simulink model "six_plus_six_AcmsteeringV09_main_1lf"  (R2014a)
settings: Solver=FixedStepDiscrete  StartTime=0.0  StopTime=10.0  FixedStep=0.0005  RelTol=1e-3
InitFcn:
  | Veh_Par_wxt
undefined symbols (not defined in the file or in its folder): acc_spdctl, ag_thr, B, bra_em, bra_pre_gz2, bra_pre_gz34, bra_pre_yd, brakepre_dem_data, brakeTrq_dem_data, bratrq_max, ecucoder_acal, eff_tran, ESP_switch, G, guzhang_lf, guzhang_lm, guzhang_lr, guzhang_rf, guzhang_rm, guzhang_rr, kd1, kd2, ki1, ki2, kp1, kp2, L, myFIS, premax, Radius, RC_switch, s_opt_yi, s_opt_zhuan, s_opt_zhuan_add, s_opt_zhuan_table, spd_map_mot, spd_spdctl, speed_thr_park, TCS_switch, tras_ratio, trq_map_mot, trqmax_yd, trqmax_zx, trqmaxneg, v_gain, v_table, v_thr_park, zhidong_bianmazhi, zhidong_down, zhidong_up, zhidong_youmen, zhuanxiang_bianmazhi, zhuanxiang_down, zhuanxiang_up, zhuanxiang_youmen
libraries: simulink x980, ec5744lib x59, fuzblock x2
(part 17 of 25)

== system six_plus_six_AcmsteeringV09_main_1lf/MainControl/mode_control/emergency_stop/emergency_stop ==
  Signals : Inport
  1-D Lookup Table : Lookup_n-D  NumberOfTableDimensions=1  BreakpointsForDimension1=zhuanxiang_youmen  Table=zhuanxiang_bianmazhi  InternalRulePriority=Speed  RndMeth=Simplest  InputSameDT=on
  1-D Lookup Table1 : Lookup_n-D  NumberOfTableDimensions=1  BreakpointsForDimension1=zhidong_youmen  Table=zhidong_bianmazhi  InternalRulePriority=Speed  RndMeth=Simplest  InputSameDT=on
  Bus Selector1 : BusSelector  OutputSignals=RemoteControl_dem.steer_dem
  Constant : Constant  Value=bra_em  OutDataTypeStr=single  SampleTime=-1
  Gain : Gain  Gain=0.5
  Gain1 : Gain  Gain=-1
  HeartBeat : MATLAB Function  TreatAsAtomicUnit=on
  HeartBeat1 : MATLAB Function  TreatAsAtomicUnit=on
  HeartBeat2 : MATLAB Function  TreatAsAtomicUnit=on
  HeartBeat3 : MATLAB Function  TreatAsAtomicUnit=on
  HeartBeat4 : MATLAB Function  TreatAsAtomicUnit=on
  HeartBeat5 : MATLAB Function  TreatAsAtomicUnit=on
  Memory{,1..4,6} (6 alike) : Memory  InheritSampleTime=on
  Mux{,1..5} (6 alike) : Mux  Inputs=6
  Saturation : Saturate  UpperLimit=zhuanxiang_up  LowerLimit=zhuanxiang_down
  Saturation2 : Saturate  UpperLimit=zhuanxiang_up  LowerLimit=zhuanxiang_down
  Saturation3 : Saturate  UpperLimit=zhuanxiang_up  LowerLimit=zhuanxiang_down
  Saturation5 : Saturate  UpperLimit=zhidong_up  LowerLimit=zhidong_down
  SpdSet_dem{,1..5} (6 alike) : Constant  Value=0  OutDataTypeStr=single  SampleTime=-1
  TrqSet_dem{,1..5} (6 alike) : Constant  Value=0  OutDataTypeStr=single  SampleTime=-1
  mot_enable{,1..5} (6 alike) : Constant  Value=0  OutDataTypeStr=single  SampleTime=-1
  mot_gear{,1..5} (6 alike) : Constant  Value=0  OutDataTypeStr=single  SampleTime=-1
  mot_mode{,1..5} (6 alike) : Constant  Value=0  OutDataTypeStr=single  SampleTime=-1
  mot_lf : Outport
  mot_lm : Outport  Port=2
  mot_lr : Outport  Port=3
  mot_rf : Outport  Port=4
  mot_rm : Outport  Port=5
  mot_rr : Outport  Port=6
  motec_position_1 : Outport  Port=7
  motec_position_2 : Outport  Port=8
  motec_position_3 : Outport  Port=9
  motec_position_4 : Outport  Port=10
  wires:
  mot_gear/1 -> Mux/3
  mot_mode/1 -> Mux/2
  SpdSet_dem/1 -> Mux/4
  TrqSet_dem/1 -> Mux/5
  Mux/1 -> mot_lf/1
  HeartBeat/1(life) -> Mux/6, Memory/1
  Memory/1 -> HeartBeat/1(life_pre)
  mot_enable/1 -> Mux/1
  mot_gear1/1 -> Mux2/3
  mot_mode2/1 -> Mux2/2
  SpdSet_dem1/1 -> Mux2/4
  TrqSet_dem1/1 -> Mux2/5
  Mux2/1 -> mot_rf/1
  HeartBeat2/1(life) -> Memory2/1, Mux2/6
  Memory2/1 -> HeartBeat2/1(life_pre)
  mot_enable1/1 -> Mux2/1
  mot_gear2/1 -> Mux4/3
  mot_mode4/1 -> Mux4/2
  SpdSet_dem4/1 -> Mux4/4
  TrqSet_dem4/1 -> Mux4/5
  Mux4/1 -> mot_lm/1
  HeartBeat3/1(life) -> Memory4/1, Mux4/6
  Memory4/1 -> HeartBeat3/1(life_pre)
  mot_enable3/1 -> Mux4/1
  mot_gear3/1 -> Mux5/3
  mot_mode5/1 -> Mux5/2
  SpdSet_dem5/1 -> Mux5/4
  TrqSet_dem5/1 -> Mux5/5
  Mux5/1 -> mot_rm/1
  HeartBeat4/1(life) -> Mux5/6, Memory6/1
  Memory6/1 -> HeartBeat4/1(life_pre)
  mot_enable5/1 -> Mux5/1
  mot_gear4/1 -> Mux1/3
  mot_mode1/1 -> Mux1/2
  SpdSet_dem2/1 -> Mux1/4
  TrqSet_dem2/1 -> Mux1/5
  Mux1/1 -> mot_lr/1
  HeartBeat1/1(life) -> Memory1/1, Mux1/6
  Memory1/1 -> HeartBeat1/1(life_pre)
  mot_enable4/1 -> Mux1/1
  mot_gear5/1 -> Mux3/3
  mot_mode3/1 -> Mux3/2
  SpdSet_dem3/1 -> Mux3/4
  TrqSet_dem3/1 -> Mux3/5
  Mux3/1 -> mot_rr/1
  HeartBeat5/1(life) -> Memory3/1, Mux3/6
  Memory3/1 -> HeartBeat5/1(life_pre)
  mot_enable2/1 -> Mux3/1
  1-D Lookup Table1/1 -> Saturation5/1
  1-D Lookup Table/1 -> Gain1/1, Gain/1, Saturation/1
  Signals/1 -> Bus Selector1/1
  Gain1/1 -> Saturation3/1
  Bus Selector1/1 -> 1-D Lookup Table/1  "<steer_dem>"
  Gain/1 -> Saturation2/1
  Saturation/1 -> motec_position_1/1
  Saturation2/1 -> motec_position_2/1
  Saturation3/1 -> motec_position_3/1
  Saturation5/1 -> motec_position_4/1
  Constant/1 -> 1-D Lookup Table1/1

== system six_plus_six_AcmsteeringV09_main_1lf/MainControl/mode_control/forward/forward ==
  Signals : Inport
  Brake : Subsystem  TreatAsAtomicUnit=on
  Bus Selector : BusSelector  OutputSignals=RemoteControl_dem.acc_dem,RemoteControl_dem.brake_dem,RemoteControl_dem.HAC
  Drive : Subsystem  TreatAsAtomicUnit=on
  MATLAB Function : MATLAB Function  TreatAsAtomicUnit=on
  Multiport Switch : MultiPortSwitch  DataPortOrder=Zero-based contiguous  Inputs=2
  Switch Case1 : SwitchCase  CaseConditions={0,1}  ShowDefaultCase=off
  forward_dem : Outport
  wires:
  Signals/1 -> Brake/1(Signals), Drive/1(Signals), Bus Selector/1
  Multiport Switch/1 -> forward_dem/1
  Switch Case1/1 -> Drive/Action
  Switch Case1/2 -> Brake/Action
  Bus Selector/1 -> MATLAB Function/1(acc_dem)  "<acc_dem>"
  MATLAB Function/1(y) -> Multiport Switch/1, Switch Case1/1
  Drive/1(forward_dem) -> Multiport Switch/2
  Brake/1(forward_dem) -> Multiport Switch/3
  Bus Selector/2 -> MATLAB Function/2(brake_dem)  "<brake_dem>"
  Bus Selector/3 -> MATLAB Function/3(HAC)  "<HAC>"

== matlab function six_plus_six_AcmsteeringV09_main_1lf/MainControl/mode_control/Park/park/HeartBeat3 ==
  data: life_pre input; life output
function life = fcn(life_pre)
%#codegen
life=single(life_pre+1);
if life>255
    life=single(0);
end
end

== system six_plus_six_AcmsteeringV09_main_1lf/MainControl/mode_control/neutral/neutral ==
  Signals : Inport
  1-D Lookup Table1 : Lookup_n-D  NumberOfTableDimensions=1  BreakpointsForDimension1=zhuanxiang_youmen  Table=zhuanxiang_bianmazhi  InternalRulePriority=Speed  RndMeth=Simplest  InputSameDT=on
  1-D Lookup Table2 : Lookup_n-D  NumberOfTableDimensions=1  BreakpointsForDimension1=zhidong_youmen  Table=zhidong_bianmazhi  InternalRulePriority=Speed  RndMeth=Simplest  InputSameDT=on
  Bus Selector : BusSelector  OutputSignals=RemoteControl_dem.steer_dem,RemoteControl_dem.brake_dem
  Gain : Gain  Gain=0.5
  Gain1 : Gain  Gain=-1
  HeartBeat : MATLAB Function  TreatAsAtomicUnit=on
  HeartBeat1 : MATLAB Function  TreatAsAtomicUnit=on
  HeartBeat2 : MATLAB Function  TreatAsAtomicUnit=on
  HeartBeat3 : MATLAB Function  TreatAsAtomicUnit=on
  HeartBeat4 : MATLAB Function  TreatAsAtomicUnit=on
  HeartBeat5 : MATLAB Function  TreatAsAtomicUnit=on
  Memory{,1..4,6} (6 alike) : Memory  InheritSampleTime=on
  Mux{,1..5} (6 alike) : Mux  Inputs=6
  Saturation : Saturate  UpperLimit=zhuanxiang_up  LowerLimit=zhuanxiang_down
  Saturation1 : Saturate  UpperLimit=zhuanxiang_up  LowerLimit=zhuanxiang_down
  Saturation2 : Saturate  UpperLimit=zhuanxiang_up  LowerLimit=zhuanxiang_down
  Saturation3 : Saturate  UpperLimit=zhidong_up  LowerLimit=zhidong_down
  SpdSet_dem{,1..5} (6 alike) : Constant  Value=0  OutDataTypeStr=single  SampleTime=-1
  TrqSet_dem{,1..5} (6 alike) : Constant  Value=0  OutDataTypeStr=single  SampleTime=-1
  mot_enable{,1..5} (6 alike) : Constant  Value=0  OutDataTypeStr=single  SampleTime=-1
  mot_gear{,1..5} (6 alike) : Constant  Value=0  OutDataTypeStr=single  SampleTime=-1
  mot_mode{,1..5} (6 alike) : Constant  Value=0  OutDataTypeStr=single  SampleTime=-1
  mot_lf : Outport
  mot_lm : Outport  Port=2
  mot_lr : Outport  Port=3
  mot_rf : Outport  Port=4
  mot_rm : Outport  Port=5
  mot_rr : Outport  Port=6
  motec_position_1 : Outport  Port=7
  motec_position_2 : Outport  Port=8
  motec_position_3 : Outport  Port=9
  motec_position_4 : Outport  Port=10
  wires:
  mot_gear/1 -> Mux/3
  mot_mode/1 -> Mux/2
  SpdSet_dem/1 -> Mux/4
  TrqSet_dem/1 -> Mux/5
  Mux/1 -> mot_lf/1
  HeartBeat/1(life) -> Mux/6, Memory/1
  Memory/1 -> HeartBeat/1(life_pre)
  mot_enable/1 -> Mux/1
  mot_gear1/1 -> Mux2/3
  mot_mode2/1 -> Mux2/2
  SpdSet_dem1/1 -> Mux2/4
  TrqSet_dem1/1 -> Mux2/5
  Mux2/1 -> mot_rf/1
  HeartBeat2/1(life) -> Memory2/1, Mux2/6
  Memory2/1 -> HeartBeat2/1(life_pre)
  mot_enable1/1 -> Mux2/1
  mot_gear2/1 -> Mux4/3
  mot_mode4/1 -> Mux4/2
  SpdSet_dem4/1 -> Mux4/4
  TrqSet_dem4/1 -> Mux4/5
  Mux4/1 -> mot_lm/1
  HeartBeat3/1(life) -> Memory4/1, Mux4/6
  Memory4/1 -> HeartBeat3/1(life_pre)
  mot_enable3/1 -> Mux4/1
  mot_gear3/1 -> Mux5/3
  mot_mode5/1 -> Mux5/2
  SpdSet_dem5/1 -> Mux5/4
  TrqSet_dem5/1 -> Mux5/5
  Mux5/1 -> mot_rm/1
  HeartBeat4/1(life) -> Mux5/6, Memory6/1
  Memory6/1 -> HeartBeat4/1(life_pre)
  mot_enable5/1 -> Mux5/1
  mot_gear4/1 -> Mux1/3
  mot_mode1/1 -> Mux1/2
  SpdSet_dem2/1 -> Mux1/4
  TrqSet_dem2/1 -> Mux1/5
  Mux1/1 -> mot_lr/1
  HeartBeat1/1(life) -> Memory1/1, Mux1/6
  Memory1/1 -> HeartBeat1/1(life_pre)
  mot_enable4/1 -> Mux1/1
  mot_gear5/1 -> Mux3/3
  mot_mode3/1 -> Mux3/2
  SpdSet_dem3/1 -> Mux3/4
  TrqSet_dem3/1 -> Mux3/5
  Mux3/1 -> mot_rr/1
  HeartBeat5/1(life) -> Memory3/1, Mux3/6
  Memory3/1 -> HeartBeat5/1(life_pre)
  mot_enable2/1 -> Mux3/1
  1-D Lookup Table1/1 -> Gain1/1, Gain/1, Saturation/1
  Signals/1 -> Bus Selector/1
  Gain1/1 -> Saturation2/1
  Bus Selector/1 -> 1-D Lookup Table1/1  "<steer_dem>"
  Gain/1 -> Saturation1/1
  Saturation/1 -> motec_position_1/1
  Saturation1/1 -> motec_position_2/1
  Saturation2/1 -> motec_position_3/1
  Saturation3/1 -> motec_position_4/1
  Bus Selector/2 -> 1-D Lookup Table2/1  "<brake_dem>"
  1-D Lookup Table2/1 -> Saturation3/1

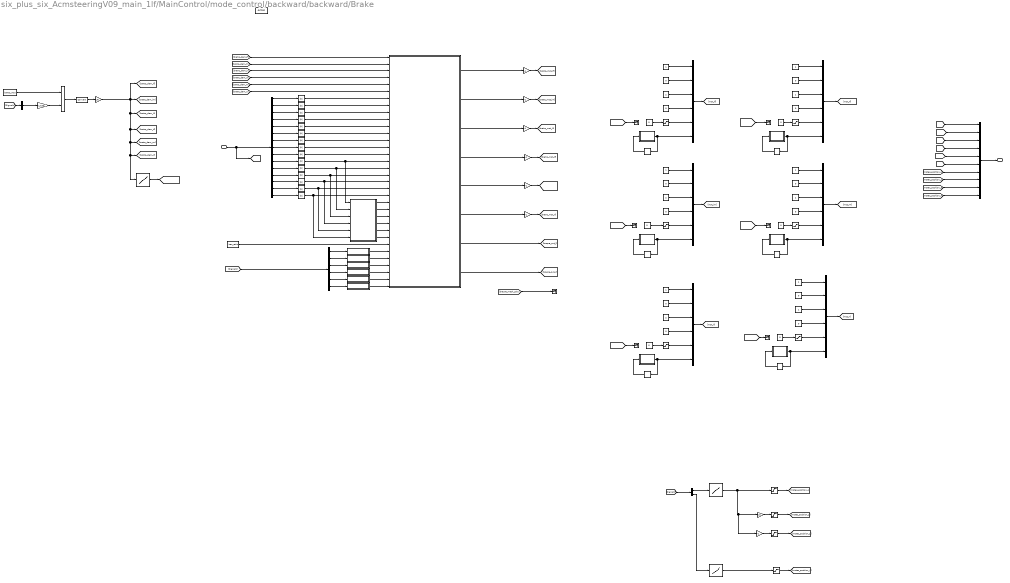
== system six_plus_six_AcmsteeringV09_main_1lf/MainControl/mode_control/backward/backward/Brake ==
  note: 当时编程序时候，fcn里面正负号搞错了，不得已在外面乘以-1，
      | 当制动时，电池功率限制，电机扭矩限制当做正值处理，电机
      | 输出力矩也是正值
  note: 制动力矩四个车轮平均分配
  Signals : Inport
  Action Port : ActionPort  ActionType=case
  1-D Lookup Table : Lookup_n-D  NumberOfTableDimensions=1  BreakpointsForDimension1=brakeTrq_dem_data  Table=brakepre_dem_data  InternalRulePriority=Speed  RndMeth=Simplest  InputSameDT=on
  1-D Lookup Table1 : Lookup_n-D  NumberOfTableDimensions=1  BreakpointsForDimension1=zhuanxiang_youmen  Table=zhuanxiang_bianmazhi  InternalRulePriority=Speed  RndMeth=Simplest  InputSameDT=on
  1-D Lookup Table2 : Lookup_n-D  NumberOfTableDimensions=1  BreakpointsForDimension1=zhidong_youmen  Table=zhidong_bianmazhi  InternalRulePriority=Speed  RndMeth=Simplest  InputSameDT=on
  Abs{1..5,10..19} (15 alike) : Abs  OutDataTypeStr=single
  Bus Selector : BusSelector  OutputSignals=RemoteControl_dem.steer_dem,RemoteControl_dem.brake_dem
  Bus Selector1 : BusSelector  OutputSignals=MOTOR.MOTOR1.MCU2,MOTOR.MOTOR3.MCU2-2,MOTOR.MOTOR5.MCU2_4,MOTOR.MOTOR2.MCU2_1,MOTOR.MOTOR4.MCU2_3,MOTOR.MOTOR6.MCU2_5
  Bus Selector2 : BusSelector  OutputSignals=RemoteControl_dem.brake_dem
  Bus Selector3 : BusSelector  OutputSignals=CCM.CCM1.BMS5.BMS5_FeedbackPower,CCM.CCM2.BMS5_1.BMS5_1FeedbackPower,CCM.CCM3.BMS5_2.BMS5_2FeedbackPower,MOTOR.MOTOR1.MCU0.MCU0_TorqueMax,MOTOR.MOTOR3.MCU0_2.MCU0_2TorqueMax,MOTOR.MOTOR5.MCU0_4.MCU0_4TorqueMax,MOTOR.MOTOR2.MCU0_1.MCU0_1TorqueMax,MOTOR.MOTOR4.MCU0_3.MCU0_3TorqueMax,MOTOR.MOTOR6.MCU0_5.MCU0_5TorqueMax,MOTOR.MOTOR1.MCU0.MCU0_SpeedFdk,MOTOR.MOTOR3.MCU0_2.MCU0_2SpeedFdk,MOTOR.MOTOR5.MCU0_4.MCU0_4SpeedFdk,MOTOR.MOTOR2.MCU0_1.MCU0_1SpeedFdk,MOTOR.MOTOR4.MCU0_3.MCU0_3SpeedFdk,MOTOR.MOTOR6.MCU0_5.MCU0_5SpeedFdk
  Constant{,1..3,5..6} (6 alike) : Constant  Value=0  SampleTime=-1
  Constant4 : Constant  Value=bratrq_max  OutDataTypeStr=single  SampleTime=-1
  Constant7 : Constant  Value=tras_ratio  OutDataTypeStr=single  SampleTime=-1
  Data Type Conversion1 : DataTypeConversion
  Gain : Gain  Gain=1/6
  Gain1 : Gain  Gain=0.5
  Gain{3,7..10,15..16} (7 alike) : Gain  Gain=-1
  Gain2 : Gain  Gain=1/100
  HeartBeat : MATLAB Function  TreatAsAtomicUnit=on
  HeartBeat1 : MATLAB Function  TreatAsAtomicUnit=on
  HeartBeat2 : MATLAB Function  TreatAsAtomicUnit=on
  HeartBeat3 : MATLAB Function  TreatAsAtomicUnit=on
  HeartBeat4 : MATLAB Function  TreatAsAtomicUnit=on
  HeartBeat5 : MATLAB Function  TreatAsAtomicUnit=on
  Memory{1..6} (6 alike) : Memory  InheritSampleTime=on
  Mux : Mux  Inputs=10
  Mux{1..6} (6 alike) : Mux  Inputs=6
  Product : Product
  Saturation{,1..5} (6 alike) : Saturate  UpperLimit=0  LowerLimit=trqmaxneg  OutDataTypeStr=single
  Saturation10 : Saturate  UpperLimit=zhuanxiang_up  LowerLimit=zhuanxiang_down
  Saturation11 : Saturate  UpperLimit=zhidong_up  LowerLimit=zhidong_down
  Saturation8 : Saturate  UpperLimit=zhuanxiang_up  LowerLimit=zhuanxiang_down
  Saturation9 : Saturate  UpperLimit=zhuanxiang_up  LowerLimit=zhuanxiang_down
  SpdSet_dem{,1..5} (6 alike) : Constant  Value=0  OutDataTypeStr=single  SampleTime=-1
  Subsystem : Subsystem
  Subsystem1 : Subsystem
  Subsystem2 : Subsystem
  Subsystem3 : Subsystem
  Subsystem4 : Subsystem
  Subsystem5 : Subsystem
  Subsystem6 : Subsystem
  Switch Case Action Subsystem : Subsystem  TreatAsAtomicUnit=on
  Terminator{,1..6} (7 alike) : Terminator
  mot_enable{1..6} (6 alike) : Constant  OutDataTypeStr=single  SampleTime=-1
  mot_gear : Constant  Value=2  OutDataTypeStr=single  SampleTime=-1
  mot_gear1 : Constant  OutDataTypeStr=single  SampleTime=-1
  mot_gear2 : Constant  Value=2  OutDataTypeStr=single  SampleTime=-1
  mot_gear3 : Constant  OutDataTypeStr=single  SampleTime=-1
  mot_gear4 : Constant  Value=2  OutDataTypeStr=single  SampleTime=-1
  mot_gear5 : Constant  OutDataTypeStr=single  SampleTime=-1
  mot_mode{,1..5} (6 alike) : Constant  Value=0  OutDataTypeStr=single  SampleTime=-1
  backward_dem : Outport
  wires:
  [Signals] -> Bus Selector2/1
  Gain/1 -> [bratrq_dem_lm], [bratrq_dem_rm], 1-D Lookup Table/1, [bratrq_dem_rr], [bratrq_dem_rf], [bratrq_dem_lr], [bratrq_dem_lf]
  Memory4/1 -> HeartBeat/1(life_pre)
  HeartBeat/1(life) -> Mux1/6, Memory4/1
  Mux1/1 -> [mot_lf]
  mot_mode/1 -> Mux1/2
  mot_gear/1 -> Mux1/3
  [mot_lf] -> Mux/1
  Signals/1 -> [Signals], Bus Selector3/1
  Constant4/1 -> Product/1
  Gain2/1 -> Product/2
  Bus Selector2/1 -> Gain2/1  "<brake_dem>"
  Product/1 -> Data Type Conversion1/1
  Gain8/1 -> [bratrq_mot_lf]
  Gain7/1 -> [bratrq_mot_lr]
  Gain9/1 -> [bratrq_mot_rf]
  Gain10/1 -> [bratrq_mot_rr]
  Constant7/1 -> Switch Case Action Subsystem/28(tras_ratio)
  1-D Lookup Table/1 -> [brapre_mech_solo]
  Data Type Conversion1/1 -> Gain/1
  Mux/1 -> backward_dem/1
  [brapre_mech_solo] -> Terminator1/1
  Switch Case Action Subsystem/1(bratrq_mot_lf) -> Gain8/1
  Gain15/1 -> [bratrq_mot_lm]
  Switch Case Action Subsystem/2(bratrq_mot_lm) -> Gain15/1
  Switch Case Action Subsystem/3(bratrq_mot_lr) -> Gain7/1
  Switch Case Action Subsystem/4(bratrq_mot_rf) -> Gain9/1
  Gain16/1 -> [bratrq_mot_rm]
  Switch Case Action Subsystem/5(bratrq_mot_rm) -> Gain16/1
  Switch Case Action Subsystem/6(bratrq_mot_rr) -> Gain10/1
  Switch Case Action Subsystem/7(brapre_out_l) -> [brapre_out_l]
  Switch Case Action Subsystem/8(brapre_out_r) -> [brapre_out_r]
  [bratrq_dem_lf] -> Switch Case Action Subsystem/1(bratrq_dem_lf)
  [bratrq_dem_rf] -> Switch Case Action Subsystem/4(bratrq_dem_rf)
  [bratrq_dem_rr] -> Switch Case Action Subsystem/6(bratrq_dem_rr)
  [bratrq_dem_lr] -> Switch Case Action Subsystem/3(bratrq_dem_lr)
  [bratrq_dem_rm] -> Switch Case Action Subsystem/5(bratrq_dem_rm)
  [bratrq_dem_lm] -> Switch Case Action Subsystem/2(bratrq_dem_lm)
  Bus Selector3/1 -> Abs5/1  "<BMS5_FeedbackPower>"
  Bus Selector3/2 -> Abs1/1  "<BMS5_1FeedbackPower>"
  Bus Selector3/3 -> Abs2/1  "<BMS5_2FeedbackPower>"
  Bus Selector3/10 -> Abs14/1  "<MCU0_SpeedFdk>"
  Bus Selector3/5 -> Abs4/1  "<MCU0_2TorqueMax>"
  Bus Selector3/7 -> Abs11/1  "<MCU0_1TorqueMax>"
  Bus Selector3/6 -> Abs10/1  "<MCU0_4TorqueMax>"
  Bus Selector3/8 -> Abs12/1  "<MCU0_3TorqueMax>"
  Bus Selector3/9 -> Abs13/1  "<MCU0_5TorqueMax>"
  Bus Selector3/4 -> Abs3/1  "<MCU0_TorqueMax>"
  Bus Selector3/11 -> Abs15/1  "<MCU0_2SpeedFdk>"
  Bus Selector3/14 -> Abs18/1  "<MCU0_3SpeedFdk>"
  Bus Selector3/12 -> Abs16/1  "<MCU0_4SpeedFdk>"
  Bus Selector3/15 -> Abs19/1  "<MCU0_5SpeedFdk>"
  Bus Selector3/13 -> Abs17/1  "<MCU0_1SpeedFdk>"
  Abs5/1 -> Switch Case Action Subsystem/7(pwr_chg_bat)
  Abs1/1 -> Switch Case Action Subsystem/8(pwr_chg_bat1)
  Abs2/1 -> Switch Case Action Subsystem/9(pwr_chg_bat2)
  Abs3/1 -> Switch Case Action Subsystem/10(trqlimL_dig_lf)
  Abs4/1 -> Switch Case Action Subsystem/11(trqlimL_dig_lm)
  Abs10/1 -> Switch Case Action Subsystem/12(trqlimL_dig_lr)
  Abs11/1 -> Switch Case Action Subsystem/13(trqlimL_dig_rf)
  Abs12/1 -> Switch Case Action Subsystem/14(trqlimL_dig_rm)
  Abs13/1 -> Switch Case Action Subsystem/15(trqlimL_dig_rr)
  Abs14/1 -> Subsystem1/1(speed_act_lf), Switch Case Action Subsystem/16(speed_act_lf)
  Abs15/1 -> Subsystem1/2(speed_act_lm), Switch Case Action Subsystem/17(speed_act_lm)
  Abs16/1 -> Subsystem1/3(speed_act_lr), Switch Case Action Subsystem/18(speed_act_lr)
  Abs17/1 -> Subsystem1/4(speed_act_rf), Switch Case Action Subsystem/19(speed_act_rf)
  Abs18/1 -> Subsystem1/5(speed_act_rm), Switch Case Action Subsystem/20(speed_act_rm)
  Abs19/1 -> Subsystem1/6(speed_act_rr), Switch Case Action Subsystem/21(speed_act_rr)
  Subsystem1/1(trqlim_map_lf) -> Switch Case Action Subsystem/22(trqlim_map_lf)
  Subsystem1/2(trqlim_map_lm) -> Switch Case Action Subsystem/23(trqlim_map_lm)
  Subsystem1/3(trqlim_map_lr) -> Switch Case Action Subsystem/24(trqlim_map_lr)
  Subsystem1/4(trqlim_map_rf) -> Switch Case Action Subsystem/25(trqlim_map_rf)
  Subsystem1/5(trqlim_map_rm) -> Switch Case Action Subsystem/26(trqlim_map_rm)
  Subsystem1/6(trqlim_map_rr) -> Switch Case Action Subsystem/27(trqlim_map_rr)
  [Signals] -> Bus Selector1/1
  Bus Selector1/1 -> Subsystem/1(MCU2)  "<MCU2>"
  Subsystem/1(guzhang_lf) -> Switch Case Action Subsystem/29(guzhang_lf)
  Bus Selector1/2 -> Subsystem2/1(MCU2_2)  "<MCU2-2>"
  Subsystem2/1(guzhang_lm) -> Switch Case Action Subsystem/30(guzhang_lm)
  Bus Selector1/3 -> Subsystem3/1(MCU2_4)  "<MCU2_4>"
  Subsystem3/1(guzhang_lr) -> Switch Case Action Subsystem/31(guzhang_lr)
  Bus Selector1/4 -> Subsystem4/1(MCU2_1)  "<MCU2_1>"
  Subsystem4/1(guzhang_rf) -> Switch Case Action Subsystem/32(guzhang_rf)
  Bus Selector1/5 -> Subsystem5/1(MCU2_3)  "<MCU2_3>"
  Subsystem5/1(guzhang_rm) -> Switch Case Action Subsystem/33(guzhang_rm)
  Bus Selector1/6 -> Subsystem6/1(MCU2_5)  "<MCU2_5>"
  Subsystem6/1(guzhang_rr) -> Switch Case Action Subsystem/34(guzhang_rr)
  mot_enable4/1 -> Mux1/1
  [bratrq_mot_lf] -> Terminator/1
  SpdSet_dem/1 -> Mux1/4
  Saturation/1 -> Mux1/5
  Memory1/1 -> HeartBeat2/1(life_pre)
  HeartBeat2/1(life) -> Memory1/1, Mux3/6
  Mux3/1 -> [mot_rf]
  mot_mode2/1 -> Mux3/2
  mot_gear1/1 -> Mux3/3
  mot_enable2/1 -> Mux3/1
  SpdSet_dem1/1 -> Mux3/4
  Saturation2/1 -> Mux3/5
  Memory3/1 -> HeartBeat3/1(life_pre)
  HeartBeat3/1(life) -> Memory3/1, Mux5/6
  Mux5/1 -> [mot_lm]
  mot_mode4/1 -> Mux5/2
  mot_gear2/1 -> Mux5/3
  mot_enable6/1 -> Mux5/1
  SpdSet_dem4/1 -> Mux5/4
  Saturation4/1 -> Mux5/5
  Memory2/1 -> HeartBeat4/1(life_pre)
  HeartBeat4/1(life) -> Mux6/6, Memory2/1
  Mux6/1 -> [mot_rm]
  mot_mode5/1 -> Mux6/2
  mot_gear3/1 -> Mux6/3
  mot_enable5/1 -> Mux6/1
  SpdSet_dem5/1 -> Mux6/4
  Saturation5/1 -> Mux6/5
  Memory5/1 -> HeartBeat1/1(life_pre)
  HeartBeat1/1(life) -> Memory5/1, Mux2/6
  Mux2/1 -> [mot_lr]
  mot_mode1/1 -> Mux2/2
  mot_gear4/1 -> Mux2/3
  mot_enable1/1 -> Mux2/1
  SpdSet_dem2/1 -> Mux2/4
  Saturation1/1 -> Mux2/5
  Memory6/1 -> HeartBeat5/1(life_pre)
  HeartBeat5/1(life) -> Mux4/6, Memory6/1
  Mux4/1 -> [mot_rr]
  mot_mode3/1 -> Mux4/2
  mot_gear5/1 -> Mux4/3
  mot_enable3/1 -> Mux4/1
  SpdSet_dem3/1 -> Mux4/4
  Saturation3/1 -> Mux4/5
  [mot_lm] -> Mux/2
  [mot_lr] -> Mux/3
  [mot_rf] -> Mux/4
  [mot_rm] -> Mux/5
  [mot_rr] -> Mux/6
  [motec_position_1] -> Mux/7
  [motec_position_2] -> Mux/8
  [motec_position_3] -> Mux/9
  Constant/1 -> Saturation/1
  [bratrq_mot_lm] -> Terminator2/1
  Constant1/1 -> Saturation4/1
  [bratrq_mot_lr] -> Terminator3/1
  Constant2/1 -> Saturation1/1
  [bratrq_mot_rf] -> Terminator4/1
  Constant3/1 -> Saturation2/1
  [bratrq_mot_rm] -> Terminator5/1
  Constant5/1 -> Saturation5/1
  [bratrq_mot_rr] -> Terminator6/1
  Constant6/1 -> Saturation3/1
  1-D Lookup Table2/1 -> Saturation11/1
  1-D Lookup Table1/1 -> Gain3/1, Gain1/1, Saturation8/1
  [Signals] -> Bus Selector/1
  Gain3/1 -> Saturation10/1
  Bus Selector/1 -> 1-D Lookup Table1/1  "<steer_dem>"
  Gain1/1 -> Saturation9/1
  Saturation8/1 -> [motec_position_1]
  Saturation9/1 -> [motec_position_2]
  Saturation10/1 -> [motec_position_3]
  Saturation11/1 -> [motec_position_4]
  Bus Selector/2 -> 1-D Lookup Table2/1  "<brake_dem>"
  [motec_position_4] -> Mux/10

== system six_plus_six_AcmsteeringV09_main_1lf/MainControl/mode_control/backward/backward/Drive ==
  Signals : Inport
  Action Port : ActionPort  ActionType=case
  Abs{,1..24} (25 alike) : Abs  OutDataTypeStr=single
  Abs25 : Abs
  Bus Selector : BusSelector  OutputSignals=RemoteControl_dem.acc_dem,MOTOR.MOTOR1.MCU0.MCU0_TorqueMax,MOTOR.MOTOR3.MCU0_2.MCU0_2TorqueMax,MOTOR.MOTOR5.MCU0_4.MCU0_4TorqueMax,MOTOR.MOTOR2.MCU0_1.MCU0_1TorqueMax,MOTOR.MOTOR4.MCU0_3.MCU0_3TorqueMax,MOTOR.MOTOR6.MCU0_5.MCU0_5TorqueMax
  Bus Selector1 : BusSelector  OutputSignals=IMU.Yacceleration
  Bus Selector2 : BusSelector  OutputSignals=IMU.Yacceleration
  Bus Selector4 : BusSelector  OutputSignals=MOTOR.MOTOR1.MCU0.MCU0_TorqueMax,MOTOR.MOTOR3.MCU0_2.MCU0_2TorqueMax,MOTOR.MOTOR5.MCU0_4.MCU0_4TorqueMax,MOTOR.MOTOR2.MCU0_1.MCU0_1TorqueMax,MOTOR.MOTOR4.MCU0_3.MCU0_3TorqueMax,MOTOR.MOTOR6.MCU0_5.MCU0_5TorqueMax,RemoteControl_dem.steer_dem
  Bus Selector5 : BusSelector  OutputSignals=CCM.CCM1.BMS5.BMS5_15s_InstanceDisPower,CCM.CCM2.BMS5_1.BMS5_1_15s_InstanceDisPower,CCM.CCM3.BMS5_2.BMS5_2_15s_InstanceDisPower,MOTOR.MOTOR1.MCU0.MCU0_SpeedFdk,MOTOR.MOTOR3.MCU0_2.MCU0_2SpeedFdk,MOTOR.MOTOR5.MCU0_4.MCU0_4SpeedFdk,MOTOR.MOTOR2.MCU0_1.MCU0_1SpeedFdk,MOTOR.MOTOR4.MCU0_3.MCU0_3SpeedFdk,MOTOR.MOTOR6.MCU0_5.MCU0_5SpeedFdk,MOTOR.MOTOR1.MCU0.MCU0_TorqueMax,MOTOR.MOTOR3.MCU0_2.MCU0_2TorqueMax,MOTOR.MOTOR5.MCU0_4.MCU0_4TorqueMax,MOTOR.MOTOR2.MCU0_1.MCU0_1TorqueMax,MOTOR.MOTOR4.MCU0_3.MCU0_3TorqueMax,MOTOR.MOTOR6.MCU0_5.MCU0_5TorqueMax
  Bus Selector6 : BusSelector  OutputSignals=MOTOR.MOTOR1.MCU2,MOTOR.MOTOR3.MCU2-2,MOTOR.MOTOR5.MCU2_4,MOTOR.MOTOR2.MCU2_1,MOTOR.MOTOR4.MCU2_3,MOTOR.MOTOR6.MCU2_5,RemoteControl_dem.center
  Bus Selector7 : BusSelector  OutputSignals=MOTOR.MOTOR1.MCU0.MCU0_SpeedFdk,MOTOR.MOTOR3.MCU0_2.MCU0_2SpeedFdk,MOTOR.MOTOR5.MCU0_4.MCU0_4SpeedFdk,MOTOR.MOTOR2.MCU0_1.MCU0_1SpeedFdk,MOTOR.MOTOR4.MCU0_3.MCU0_3SpeedFdk,MOTOR.MOTOR6.MCU0_5.MCU0_5SpeedFdk,IMU.Xspd,RemoteControl_dem.brake_dem
  Bus Selector8 : BusSelector  OutputSignals=MOTOR.MOTOR1.MCU0.MCU0_SpeedFdk,MOTOR.MOTOR3.MCU0_2.MCU0_2SpeedFdk,MOTOR.MOTOR5.MCU0_4.MCU0_4SpeedFdk,MOTOR.MOTOR2.MCU0_1.MCU0_1SpeedFdk,MOTOR.MOTOR4.MCU0_3.MCU0_3SpeedFdk,MOTOR.MOTOR6.MCU0_5.MCU0_5SpeedFdk
  Bus Selector9 : BusSelector  OutputSignals=MOTOR.MOTOR1.MCU0.MCU0_SpeedFdk,MOTOR.MOTOR3.MCU0_2.MCU0_2SpeedFdk,MOTOR.MOTOR5.MCU0_4.MCU0_4SpeedFdk,MOTOR.MOTOR2.MCU0_1.MCU0_1SpeedFdk,MOTOR.MOTOR4.MCU0_3.MCU0_3SpeedFdk,MOTOR.MOTOR6.MCU0_5.MCU0_5SpeedFdk
  Constant1 : Constant  Value=ag_thr  OutDataTypeStr=single  SampleTime=-1
  Gain : Gain  Gain=3.6  OutDataTypeStr=single
  Ground3 : Ground
  Ground4 : Ground
  Ground5 : Ground
  MATLAB Function : MATLAB Function  TreatAsAtomicUnit=on
  Multiport Switch : MultiPortSwitch  DataPortOrder=Zero-based contiguous  Inputs=2
  Subsystem : Subsystem
  Subsystem1 : Subsystem
  Subsystem2 : Subsystem
  Subsystem3 : Subsystem
  Subsystem4 : Subsystem
  Subsystem5 : Subsystem
  Switch Case : SwitchCase  CaseConditions={0,1}  ShowDefaultCase=off
  Terminator : Terminator
  Terminator2 : Terminator
  容错控制 : Subsystem
  左右侧电机分配及功率限制 : Subsystem
  目标直驶力矩确定模块 : Subsystem
  目标转向力矩确定模块 : Subsystem  TreatAsAtomicUnit=on
  路面状况识别模块 : Subsystem
  车辆稳定性控制 : Subsystem  TreatAsAtomicUnit=on
  车辆稳定性控制1 : Subsystem  TreatAsAtomicUnit=on
  驱动防滑控制TCS : Subsystem
  backward_dem : Outport
  wires:
  [umax] -> 目标转向力矩确定模块/8(umax)
  [f] -> 目标转向力矩确定模块/9(f)
  路面状况识别模块/1(umax) -> [umax]
  路面状况识别模块/2(f) -> [f]
  路面状况识别模块/3(s_opt_zhuan) -> [s_opt_zhuan]
  目标直驶力矩确定模块/1(Trq_line_dem) -> 左右侧电机分配及功率限制/1(Trq_line_dem)
  [Signals] -> Bus Selector5/1
  [Signals] -> Bus Selector6/1
  左右侧电机分配及功率限制/2(trq_dem_r) -> 容错控制/2(trq_dem_r)
  左右侧电机分配及功率限制/1(trq_dem_l) -> 容错控制/1(trq_dem_l)
  左右侧电机分配及功率限制/6(trqlim_rf) -> 容错控制/6(trqlim_rf)
  左右侧电机分配及功率限制/5(trqlim_lr) -> 容错控制/5(trqlim_lr)
  左右侧电机分配及功率限制/8(trqlim_rr) -> 容错控制/8(trqlim_rr)
  左右侧电机分配及功率限制/3(trqlim_lf) -> 容错控制/3(trqlim_lf)
  容错控制/1(trq_dem_lf) -> 驱动防滑控制TCS/1(trq_dem_lf)
  容错控制/7(bra_pre_l) -> 驱动防滑控制TCS/7(bra_pre_l)
  容错控制/8(bra_pre_r) -> 驱动防滑控制TCS/8(bra_pre_r)
  容错控制/4(trq_dem_rf) -> 驱动防滑控制TCS/4(trq_dem_rf)
  容错控制/6(trq_dem_rr) -> 驱动防滑控制TCS/6(trq_dem_rr)
  [Signals] -> Bus Selector7/1
  驱动防滑控制TCS/1(backward_dem) -> backward_dem/1
  路面状况识别模块/4(s_opt_yi) -> Terminator/1
  [Signals] -> Bus Selector8/1
  [Signals] -> Bus Selector9/1
  容错控制/3(trq_dem_lr) -> 驱动防滑控制TCS/3(trq_dem_lr)
  Ground5/1 -> 路面状况识别模块/1(In1)
  Ground3/1 -> 路面状况识别模块/2(miu)
  Ground4/1 -> 路面状况识别模块/3(slip_ratio)
  Bus Selector/7 -> 目标直驶力矩确定模块/7(TrqLimU_dig_rr)  "<MCU0_5TorqueMax>"
  Bus Selector/6 -> 目标直驶力矩确定模块/6(TrqLimU_dig_rm)  "<MCU0_3TorqueMax>"
  Bus Selector/5 -> 目标直驶力矩确定模块/5(TrqLimU_dig_rf)  "<MCU0_1TorqueMax>"
  Bus Selector/4 -> 目标直驶力矩确定模块/4(TrqLimU_dig_lr)  "<MCU0_4TorqueMax>"
  Bus Selector/3 -> 目标直驶力矩确定模块/3(TrqLimU_dig_lm)  "<MCU0_2TorqueMax>"
  Bus Selector/2 -> 目标直驶力矩确定模块/2(TrqLimU_dig_lf)  "<MCU0_TorqueMax>"
  Bus Selector/1 -> Abs25/1  "<acc_dem>"
  Abs12/1 -> 目标直驶力矩确定模块/9(speed_act_lm)
  Abs11/1 -> 目标直驶力矩确定模块/8(speed_act_lf)
  Abs13/1 -> 目标直驶力矩确定模块/10(speed_act_lr)
  Abs14/1 -> 目标直驶力矩确定模块/11(speed_act_rf)
  Abs19/1 -> 目标直驶力矩确定模块/12(speed_act_rm)
  Abs20/1 -> 目标直驶力矩确定模块/13(speed_act_rr)
  Bus Selector4/7 -> 目标转向力矩确定模块/7(steer_dem)  "<steer_dem>"
  Abs15/1 -> 目标转向力矩确定模块/10(speed_act_lf)
  Abs16/1 -> 目标转向力矩确定模块/11(speed_act_lm)
  Abs17/1 -> 目标转向力矩确定模块/12(speed_act_lr)
  Abs18/1 -> 目标转向力矩确定模块/13(speed_act_rf)
  Abs21/1 -> 目标转向力矩确定模块/14(speed_act_rm)
  Abs22/1 -> 目标转向力矩确定模块/15(speed_act_rr)
  Bus Selector5/2 -> 左右侧电机分配及功率限制/4(pwr_dis_bat1)  "<BMS5_1_15s_InstanceDisPower>"
  Bus Selector5/3 -> 左右侧电机分配及功率限制/5(pwr_dis_bat2)  "<BMS5_2_15s_InstanceDisPower>"
  Bus Selector5/1 -> 左右侧电机分配及功率限制/3(pwr_dis_bat)  "<BMS5_15s_InstanceDisPower>"
  Abs/1 -> 左右侧电机分配及功率限制/6(speed_act_lf)
  Abs1/1 -> 左右侧电机分配及功率限制/7(speed_act_lm)
  Abs10/1 -> 左右侧电机分配及功率限制/8(speed_act_lr)
  Abs2/1 -> 左右侧电机分配及功率限制/9(speed_act_rf)
  Abs24/1 -> 左右侧电机分配及功率限制/10(speed_act_rm)
  Abs3/1 -> 左右侧电机分配及功率限制/11(speed_act_rr)
  左右侧电机分配及功率限制/4(trqlim_lm) -> 容错控制/4(trqlim_lm)
  容错控制/2(trq_dem_lm) -> 驱动防滑控制TCS/2(trq_dem_lm)
  容错控制/5(trq_dem_rm) -> 驱动防滑控制TCS/5(trq_dem_rm)
  左右侧电机分配及功率限制/7(trqlim_rm) -> 容错控制/7(trqlim_rm)
  Bus Selector6/1 -> Subsystem/1(MCU2)  "<MCU2>"
  Subsystem/1(guzhang_lf) -> 容错控制/9(guzhang_lf)
  Bus Selector6/2 -> Subsystem1/1(MCU2_2)  "<MCU2-2>"
  Subsystem1/1(guzhang_lm) -> 容错控制/10(guzhang_lm)
  Bus Selector6/3 -> Subsystem2/1(MCU2_4)  "<MCU2_4>"
  Subsystem2/1(guzhang_lr) -> 容错控制/11(guzhang_lr)
  Bus Selector6/4 -> Subsystem3/1(MCU2_1)  "<MCU2_1>"
  Subsystem3/1(guzhang_rf) -> 容错控制/12(guzhang_rf)
  Bus Selector6/5 -> Subsystem4/1(MCU2_3)  "<MCU2_3>"
  Subsystem4/1(guzhang_rm) -> 容错控制/13(guzhang_rm)
  Bus Selector6/6 -> Subsystem5/1(MCU2_5)  "<MCU2_5>"
  Subsystem5/1(guzhang_rr) -> 容错控制/14(guzhang_rr)
  Bus Selector8/2 -> Abs12/1  "<MCU0_2SpeedFdk>"
  Bus Selector8/1 -> Abs11/1  "<MCU0_SpeedFdk>"
  Bus Selector8/3 -> Abs13/1  "<MCU0_4SpeedFdk>"
  Bus Selector8/4 -> Abs14/1  "<MCU0_1SpeedFdk>"
  Bus Selector8/5 -> Abs19/1  "<MCU0_3SpeedFdk>"
  Bus Selector8/6 -> Abs20/1  "<MCU0_5SpeedFdk>"
  Bus Selector4/1 -> 目标转向力矩确定模块/1(TrqLimU_dig_lf)  "<MCU0_TorqueMax>"
  Bus Selector4/2 -> 目标转向力矩确定模块/2(TrqLimU_dig_lm)  "<MCU0_2TorqueMax>"
  Bus Selector4/5 -> 目标转向力矩确定模块/5(TrqLimU_dig_rm)  "<MCU0_3TorqueMax>"
  Bus Selector4/6 -> 目标转向力矩确定模块/6(TrqLimU_dig_rr)  "<MCU0_5TorqueMax>"
  Bus Selector4/3 -> 目标转向力矩确定模块/3(TrqLimU_dig_lr)  "<MCU0_4TorqueMax>"
  Bus Selector4/4 -> 目标转向力矩确定模块/4(TrqLimU_dig_rf)  "<MCU0_1TorqueMax>"
  Bus Selector9/2 -> Abs16/1  "<MCU0_2SpeedFdk>"
  Bus Selector9/3 -> Abs17/1  "<MCU0_4SpeedFdk>"
  Bus Selector9/4 -> Abs18/1  "<MCU0_1SpeedFdk>"
  Bus Selector9/1 -> Abs15/1  "<MCU0_SpeedFdk>"
  Bus Selector9/5 -> Abs21/1  "<MCU0_3SpeedFdk>"
  Bus Selector9/6 -> Abs22/1  "<MCU0_5SpeedFdk>"
  Bus Selector5/5 -> Abs1/1  "<MCU0_2SpeedFdk>"
  Bus Selector5/4 -> Abs/1  "<MCU0_SpeedFdk>"
  Bus Selector5/9 -> Abs3/1  "<MCU0_5SpeedFdk>"
  Bus Selector5/7 -> Abs2/1  "<MCU0_1SpeedFdk>"
  Bus Selector5/6 -> Abs10/1  "<MCU0_4SpeedFdk>"
  Bus Selector5/8 -> Abs24/1  "<MCU0_3SpeedFdk>"
  Bus Selector5/15 -> 左右侧电机分配及功率限制/17(TrqLimU_dig_rr)  "<MCU0_5TorqueMax>"
  Bus Selector5/14 -> 左右侧电机分配及功率限制/16(TrqLimU_dig_rm)  "<MCU0_3TorqueMax>"
  Bus Selector5/11 -> 左右侧电机分配及功率限制/13(TrqLimU_dig_lm)  "<MCU0_2TorqueMax>"
  Bus Selector5/12 -> 左右侧电机分配及功率限制/14(TrqLimU_dig_lr)  "<MCU0_4TorqueMax>"
  Bus Selector5/13 -> 左右侧电机分配及功率限制/15(TrqLimU_dig_rf)  "<MCU0_1TorqueMax>"
  Bus Selector5/10 -> 左右侧电机分配及功率限制/12(TrqLimU_dig_lf)  "<MCU0_TorqueMax>"
  目标转向力矩确定模块/1(delta_Tsteer_dem) -> Terminator2/1
  Bus Selector7/1 -> Abs4/1  "<MCU0_SpeedFdk>"
  Bus Selector7/2 -> Abs5/1  "<MCU0_2SpeedFdk>"
  Bus Selector7/3 -> Abs6/1  "<MCU0_4SpeedFdk>"
  Bus Selector7/4 -> Abs7/1  "<MCU0_1SpeedFdk>"
  Bus Selector7/5 -> Abs8/1  "<MCU0_3SpeedFdk>"
  Bus Selector7/6 -> Abs9/1  "<MCU0_5SpeedFdk>"
  Bus Selector7/7 -> Gain/1  "<Xspd>"
  Bus Selector7/8 -> 驱动防滑控制TCS/16(brake_dem)  "<brake_dem>"
  [s_opt_zhuan] -> 驱动防滑控制TCS/17(s_opt_zhuan)
  Abs4/1 -> 驱动防滑控制TCS/9(speed_act_lf)
  Abs5/1 -> 驱动防滑控制TCS/10(speed_act_lm)
  Abs6/1 -> 驱动防滑控制TCS/11(speed_act_lr)
  Abs7/1 -> 驱动防滑控制TCS/12(speed_act_rf)
  Abs8/1 -> 驱动防滑控制TCS/13(speed_act_rm)
  Abs9/1 -> 驱动防滑控制TCS/14(speed_act_rr)
  Abs23/1 -> 驱动防滑控制TCS/15(v_act)
  [Signals] -> 驱动防滑控制TCS/18(Signals)
  Abs25/1 -> 目标直驶力矩确定模块/1(acc_dem)
  Gain/1 -> Abs23/1
  [Signals] -> 路面状况识别模块/4(Signals)
  Signals/1 -> Bus Selector2/1, Bus Selector4/1, Bus Selector1/1, [Signals], Bus Selector/1
  Bus Selector1/1 -> 车辆稳定性控制/1(acc_y)  "<Yacceleration>"
  车辆稳定性控制/1(delta_Twending_dem) -> Multiport Switch/2
  MATLAB Function/1(y) -> Multiport Switch/1, Switch Case/1
  Switch Case/2 -> 车辆稳定性控制1/Action
  Switch Case/1 -> 车辆稳定性控制/Action
  Constant1/1 -> MATLAB Function/2(ag_thr)
  Multiport Switch/1 -> 左右侧电机分配及功率限制/2(delta_T_dem)
  Bus Selector2/1 -> MATLAB Function/1(acc_y)  "<Yacceleration>"
  车辆稳定性控制1/1(1) -> Multiport Switch/3
  Bus Selector6/7 -> 容错控制/15(guzhang_flag)  "<center>"

== system six_plus_six_AcmsteeringV09_main_1lf/MainControl/mode_control/center_steer/center_steer/Subsystem ==
  MCU2 : Inport
  Bus Selector : BusSelector  OutputSignals=MCU2_MotorStallingFault,MCU2_UdcDetectionFault,MCU2_TempSensorFault,MCU2_ActiveDischargingFault,MCU2_ldcSensorFault,MCU2_luSensorFault,MCU2_lvSensorFault,MCU2_FaultLevel,MCU2_Controllerload,MCU2_CanCommunicationFault,MCU2_MemoryFault,MCU2_DownratingFault,MCU2_IGBTFault,MCU2_MotorOverTemp,MCU2_ControllerOverTemp,MCU2_MotorOverSpeed,MCU2_RotaryInverterFault,MCU2_UnderVoltage,MCU2_OverVoltage,MCU2_MotorOverLoad
  Compare To Constant{,1..19} (20 alike) : simulink/Logic and Bit Operations/Compare To Constant  relop===  const=1  OutDataTypeStr=boolean
  Logical Operator : Logic  Operator=OR  Inputs=20  AllPortsSameDT=off  OutDataTypeStr=boolean
  guzhang_lf : Outport
  wires:
  MCU2/1 -> Bus Selector/1
  Bus Selector/1 -> Compare To Constant/1  "<MCU2_MotorStallingFault>"
  Bus Selector/2 -> Compare To Constant1/1  "<MCU2_UdcDetectionFault>"
  Bus Selector/3 -> Compare To Constant2/1  "<MCU2_TempSensorFault>"
  Bus Selector/4 -> Compare To Constant3/1  "<MCU2_ActiveDischargingFault>"
  Bus Selector/5 -> Compare To Constant4/1  "<MCU2_ldcSensorFault>"
  Bus Selector/6 -> Compare To Constant5/1  "<MCU2_luSensorFault>"
  Bus Selector/7 -> Compare To Constant6/1  "<MCU2_lvSensorFault>"
  Bus Selector/8 -> Compare To Constant7/1  "<MCU2_FaultLevel>"
  Bus Selector/13 -> Compare To Constant12/1  "<MCU2_IGBTFault>"
  Bus Selector/14 -> Compare To Constant13/1  "<MCU2_MotorOverTemp>"
  Bus Selector/10 -> Compare To Constant9/1  "<MCU2_CanCommunicationFault>"
  Bus Selector/16 -> Compare To Constant15/1  "<MCU2_MotorOverSpeed>"
  Bus Selector/11 -> Compare To Constant10/1  "<MCU2_MemoryFault>"
  Bus Selector/15 -> Compare To Constant14/1  "<MCU2_ControllerOverTemp>"
  Bus Selector/12 -> Compare To Constant11/1  "<MCU2_DownratingFault>"
  Bus Selector/9 -> Compare To Constant8/1  "<MCU2_Controllerload>"
  Bus Selector/18 -> Compare To Constant17/1  "<MCU2_UnderVoltage>"
  Bus Selector/20 -> Compare To Constant19/1  "<MCU2_MotorOverLoad>"
  Bus Selector/19 -> Compare To Constant18/1  "<MCU2_OverVoltage>"
  Bus Selector/17 -> Compare To Constant16/1  "<MCU2_RotaryInverterFault>"
  Compare To Constant9/1 -> Logical Operator/10
  Compare To Constant12/1 -> Logical Operator/13
  Compare To Constant11/1 -> Logical Operator/12
  Compare To Constant15/1 -> Logical Operator/16
  Compare To Constant8/1 -> Logical Operator/9
  Compare To Constant10/1 -> Logical Operator/11
  Compare To Constant13/1 -> Logical Operator/14
  Compare To Constant14/1 -> Logical Operator/15
  Compare To Constant1/1 -> Logical Operator/2
  Compare To Constant17/1 -> Logical Operator/18
  Compare To Constant16/1 -> Logical Operator/17
  Compare To Constant18/1 -> Logical Operator/19
  Compare To Constant19/1 -> Logical Operator/20
  Compare To Constant3/1 -> Logical Operator/4
  Compare To Constant2/1 -> Logical Operator/3
  Compare To Constant6/1 -> Logical Operator/7
  Compare To Constant4/1 -> Logical Operator/5
  Compare To Constant5/1 -> Logical Operator/6
  Compare To Constant7/1 -> Logical Operator/8
  Compare To Constant/1 -> Logical Operator/1
  Logical Operator/1 -> guzhang_lf/1

== system six_plus_six_AcmsteeringV09_main_1lf/MainControl/mode_control/center_steer/center_steer/Subsystem1 ==
  MCU2_2 : Inport
  Bus Selector : BusSelector  OutputSignals=MCU2_2MotorStallingFault,MCU2_2UdcDetectionFault,MCU2_2TempSensorFault,MCU2_2ActiveDischargingFault,MCU2_2ldcSensorFault,MCU2_2luSensorFault,MCU2_2lvSensorFault,MCU2_2FaultLevel,MCU2_2Controllerload,MCU2_2CanCommunicationFault,MCU2_2MemoryFault,MCU2_2DownratingFault,MCU2_2IGBTFault,MCU2_2MotorOverTemp,MCU2_2ControllerOverTemp,MCU2_2MotorOverSpeed,MCU2_2RotaryInverterFault,MCU2_2UnderVoltage,MCU2_OverVoltage,MCU2_2MotorOverLoad
  Compare To Constant{,1..19} (20 alike) : simulink/Logic and Bit Operations/Compare To Constant  relop===  const=1  OutDataTypeStr=boolean
  Logical Operator : Logic  Operator=OR  Inputs=20  AllPortsSameDT=off  OutDataTypeStr=boolean
  guzhang_lm : Outport
  wires:
  Logical Operator/1 -> guzhang_lm/1
  Compare To Constant/1 -> Logical Operator/1
  Compare To Constant7/1 -> Logical Operator/8
  Compare To Constant5/1 -> Logical Operator/6
  Compare To Constant4/1 -> Logical Operator/5
  Compare To Constant6/1 -> Logical Operator/7
  Compare To Constant2/1 -> Logical Operator/3
  Compare To Constant3/1 -> Logical Operator/4
  Compare To Constant19/1 -> Logical Operator/20
  Compare To Constant18/1 -> Logical Operator/19
  Compare To Constant16/1 -> Logical Operator/17
  Compare To Constant17/1 -> Logical Operator/18
  Compare To Constant1/1 -> Logical Operator/2
  Compare To Constant14/1 -> Logical Operator/15
  Compare To Constant13/1 -> Logical Operator/14
  Compare To Constant10/1 -> Logical Operator/11
  Compare To Constant8/1 -> Logical Operator/9
  Compare To Constant15/1 -> Logical Operator/16
  Compare To Constant11/1 -> Logical Operator/12
  Compare To Constant12/1 -> Logical Operator/13
  Compare To Constant9/1 -> Logical Operator/10
  Bus Selector/17 -> Compare To Constant16/1  "<MCU2_2RotaryInverterFault>"
  Bus Selector/19 -> Compare To Constant18/1  "<MCU2_OverVoltage>"
  Bus Selector/20 -> Compare To Constant19/1  "<MCU2_2MotorOverLoad>"
  Bus Selector/18 -> Compare To Constant17/1  "<MCU2_2UnderVoltage>"
  Bus Selector/9 -> Compare To Constant8/1  "<MCU2_2Controllerload>"
  Bus Selector/12 -> Compare To Constant11/1  "<MCU2_2DownratingFault>"
  Bus Selector/15 -> Compare To Constant14/1  "<MCU2_2ControllerOverTemp>"
  Bus Selector/11 -> Compare To Constant10/1  "<MCU2_2MemoryFault>"
  Bus Selector/16 -> Compare To Constant15/1  "<MCU2_2MotorOverSpeed>"
  Bus Selector/10 -> Compare To Constant9/1  "<MCU2_2CanCommunicationFault>"
  Bus Selector/14 -> Compare To Constant13/1  "<MCU2_2MotorOverTemp>"
  Bus Selector/13 -> Compare To Constant12/1  "<MCU2_2IGBTFault>"
  Bus Selector/8 -> Compare To Constant7/1  "<MCU2_2FaultLevel>"
  Bus Selector/7 -> Compare To Constant6/1  "<MCU2_2lvSensorFault>"
  Bus Selector/6 -> Compare To Constant5/1  "<MCU2_2luSensorFault>"
  Bus Selector/5 -> Compare To Constant4/1  "<MCU2_2ldcSensorFault>"
  Bus Selector/4 -> Compare To Constant3/1  "<MCU2_2ActiveDischargingFault>"
  Bus Selector/3 -> Compare To Constant2/1  "<MCU2_2TempSensorFault>"
  Bus Selector/2 -> Compare To Constant1/1  "<MCU2_2UdcDetectionFault>"
  Bus Selector/1 -> Compare To Constant/1  "<MCU2_2MotorStallingFault>"
  MCU2_2/1 -> Bus Selector/1

== system six_plus_six_AcmsteeringV09_main_1lf/MainControl/mode_control/center_steer/center_steer/Subsystem2 ==
  MCU2_4 : Inport
  Bus Selector : BusSelector  OutputSignals=MCU2_4MotorStallingFault,MCU2_4UdcDetectionFault,MCU2_4TempSensorFault,MCU2_4ActiveDischargingFault,MCU2_4ldcSensorFault,MCU2_4luSensorFault,MCU2_4lvSensorFault,MCU2_4FaultLevel,MCU2_4Controllerload,MCU2_4CanCommunicationFault,MCU2_4MemoryFault,MCU2_4DownratingFault,MCU2_4IGBTFault,MCU2_4MotorOverTemp,MCU2_4ControllerOverTemp,MCU2_4MotorOverSpeed,MCU2_4RotaryInverterFault,MCU2_4UnderVoltage,MCU2_4OverVoltage,MCU2_4MotorOverLoad
  Compare To Constant{,1..19} (20 alike) : simulink/Logic and Bit Operations/Compare To Constant  relop===  const=1  OutDataTypeStr=boolean
  Logical Operator : Logic  Operator=OR  Inputs=20  AllPortsSameDT=off  OutDataTypeStr=boolean
  guzhang_lr : Outport
  wires:
  MCU2_4/1 -> Bus Selector/1
  Bus Selector/1 -> Compare To Constant/1  "<MCU2_4MotorStallingFault>"
  Bus Selector/2 -> Compare To Constant1/1  "<MCU2_4UdcDetectionFault>"
  Bus Selector/3 -> Compare To Constant2/1  "<MCU2_4TempSensorFault>"
  Bus Selector/4 -> Compare To Constant3/1  "<MCU2_4ActiveDischargingFault>"
  Bus Selector/5 -> Compare To Constant4/1  "<MCU2_4ldcSensorFault>"
  Bus Selector/6 -> Compare To Constant5/1  "<MCU2_4luSensorFault>"
  Bus Selector/7 -> Compare To Constant6/1  "<MCU2_4lvSensorFault>"
  Bus Selector/8 -> Compare To Constant7/1  "<MCU2_4FaultLevel>"
  Bus Selector/13 -> Compare To Constant12/1  "<MCU2_4IGBTFault>"
  Bus Selector/14 -> Compare To Constant13/1  "<MCU2_4MotorOverTemp>"
  Bus Selector/10 -> Compare To Constant9/1  "<MCU2_4CanCommunicationFault>"
  Bus Selector/16 -> Compare To Constant15/1  "<MCU2_4MotorOverSpeed>"
  Bus Selector/11 -> Compare To Constant10/1  "<MCU2_4MemoryFault>"
  Bus Selector/15 -> Compare To Constant14/1  "<MCU2_4ControllerOverTemp>"
  Bus Selector/12 -> Compare To Constant11/1  "<MCU2_4DownratingFault>"
  Bus Selector/9 -> Compare To Constant8/1  "<MCU2_4Controllerload>"
  Bus Selector/18 -> Compare To Constant17/1  "<MCU2_4UnderVoltage>"
  Bus Selector/20 -> Compare To Constant19/1  "<MCU2_4MotorOverLoad>"
  Bus Selector/19 -> Compare To Constant18/1  "<MCU2_4OverVoltage>"
  Bus Selector/17 -> Compare To Constant16/1  "<MCU2_4RotaryInverterFault>"
  Compare To Constant9/1 -> Logical Operator/10
  Compare To Constant12/1 -> Logical Operator/13
  Compare To Constant11/1 -> Logical Operator/12
  Compare To Constant15/1 -> Logical Operator/16
  Compare To Constant8/1 -> Logical Operator/9
  Compare To Constant10/1 -> Logical Operator/11
  Compare To Constant13/1 -> Logical Operator/14
  Compare To Constant14/1 -> Logical Operator/15
  Compare To Constant1/1 -> Logical Operator/2
  Compare To Constant17/1 -> Logical Operator/18
  Compare To Constant16/1 -> Logical Operator/17
  Compare To Constant18/1 -> Logical Operator/19
  Compare To Constant19/1 -> Logical Operator/20
  Compare To Constant3/1 -> Logical Operator/4
  Compare To Constant2/1 -> Logical Operator/3
  Compare To Constant6/1 -> Logical Operator/7
  Compare To Constant4/1 -> Logical Operator/5
  Compare To Constant5/1 -> Logical Operator/6
  Compare To Constant7/1 -> Logical Operator/8
  Compare To Constant/1 -> Logical Operator/1
  Logical Operator/1 -> guzhang_lr/1

== system six_plus_six_AcmsteeringV09_main_1lf/MainControl/mode_control/center_steer/center_steer/Subsystem3 ==
  MCU2_1 : Inport
  Bus Selector : BusSelector  OutputSignals=MCU2_1MotorStallingFault,MCU2_1UdcDetectionFault,MCU2_1TempSensorFault,MCU2_1ActiveDischargingFault,MCU2_1ldcSensorFault,MCU2_1luSensorFault,MCU2_1lvSensorFault,MCU2_1FaultLevel,MCU2_1Controllerload,MCU2_1CanCommunicationFault,MCU2_1MemoryFault,MCU2_1DownratingFault,MCU2_1IGBTFault,MCU2_1MotorOverTemp,MCU2_1ControllerOverTemp,MCU2_1MotorOverSpeed,MCU2_1RotaryInverterFault,MCU2_1UnderVoltage,MCU2_1OverVoltage,MCU2_1MotorOverLoad
  Compare To Constant{,1..19} (20 alike) : simulink/Logic and Bit Operations/Compare To Constant  relop===  const=1  OutDataTypeStr=boolean
  Logical Operator : Logic  Operator=OR  Inputs=20  AllPortsSameDT=off  OutDataTypeStr=boolean
  guzhang_rf : Outport
  wires:
  Logical Operator/1 -> guzhang_rf/1
  Compare To Constant/1 -> Logical Operator/1
  Compare To Constant7/1 -> Logical Operator/8
  Compare To Constant5/1 -> Logical Operator/6
  Compare To Constant4/1 -> Logical Operator/5
  Compare To Constant6/1 -> Logical Operator/7
  Compare To Constant2/1 -> Logical Operator/3
  Compare To Constant3/1 -> Logical Operator/4
  Compare To Constant19/1 -> Logical Operator/20
  Compare To Constant18/1 -> Logical Operator/19
  Compare To Constant16/1 -> Logical Operator/17
  Compare To Constant17/1 -> Logical Operator/18
  Compare To Constant1/1 -> Logical Operator/2
  Compare To Constant14/1 -> Logical Operator/15
  Compare To Constant13/1 -> Logical Operator/14
  Compare To Constant10/1 -> Logical Operator/11
  Compare To Constant8/1 -> Logical Operator/9
  Compare To Constant15/1 -> Logical Operator/16
  Compare To Constant11/1 -> Logical Operator/12
  Compare To Constant12/1 -> Logical Operator/13
  Compare To Constant9/1 -> Logical Operator/10
  Bus Selector/17 -> Compare To Constant16/1  "<MCU2_1RotaryInverterFault>"
  Bus Selector/19 -> Compare To Constant18/1  "<MCU2_1OverVoltage>"
  Bus Selector/20 -> Compare To Constant19/1  "<MCU2_1MotorOverLoad>"
  Bus Selector/18 -> Compare To Constant17/1  "<MCU2_1UnderVoltage>"
  Bus Selector/9 -> Compare To Constant8/1  "<MCU2_1Controllerload>"
  Bus Selector/12 -> Compare To Constant11/1  "<MCU2_1DownratingFault>"
  Bus Selector/15 -> Compare To Constant14/1  "<MCU2_1ControllerOverTemp>"
  Bus Selector/11 -> Compare To Constant10/1  "<MCU2_1MemoryFault>"
  Bus Selector/16 -> Compare To Constant15/1  "<MCU2_1MotorOverSpeed>"
  Bus Selector/10 -> Compare To Constant9/1  "<MCU2_1CanCommunicationFault>"
  Bus Selector/14 -> Compare To Constant13/1  "<MCU2_1MotorOverTemp>"
  Bus Selector/13 -> Compare To Constant12/1  "<MCU2_1IGBTFault>"
  Bus Selector/8 -> Compare To Constant7/1  "<MCU2_1FaultLevel>"
  Bus Selector/7 -> Compare To Constant6/1  "<MCU2_1lvSensorFault>"
  Bus Selector/6 -> Compare To Constant5/1  "<MCU2_1luSensorFault>"
  Bus Selector/5 -> Compare To Constant4/1  "<MCU2_1ldcSensorFault>"
  Bus Selector/4 -> Compare To Constant3/1  "<MCU2_1ActiveDischargingFault>"
  Bus Selector/3 -> Compare To Constant2/1  "<MCU2_1TempSensorFault>"
  Bus Selector/2 -> Compare To Constant1/1  "<MCU2_1UdcDetectionFault>"
  Bus Selector/1 -> Compare To Constant/1  "<MCU2_1MotorStallingFault>"
  MCU2_1/1 -> Bus Selector/1

== system six_plus_six_AcmsteeringV09_main_1lf/MainControl/mode_control/center_steer/center_steer/Subsystem4 ==
  MCU2_3 : Inport
  Bus Selector : BusSelector  OutputSignals=MCU2_3MotorStallingFault,MCU2_3UdcDetectionFault,MCU2_3TempSensorFault,MCU2_3ActiveDischargingFault,MCU2_3ldcSensorFault,MCU2_3luSensorFault,MCU2_3lvSensorFault,MCU2_3FaultLevel,MCU2_3Controllerload,MCU2_3CanCommunicationFault,MCU2_3MemoryFault,MCU2_3DownratingFault,MCU2_3IGBTFault,MCU2_3MotorOverTemp,MCU2_3ControllerOverTemp,MCU2_3MotorOverSpeed,MCU2_3RotaryInverterFault,MCU2_3UnderVoltage,MCU2_3OverVoltage,MCU2_3MotorOverLoad
  Compare To Constant{,1..19} (20 alike) : simulink/Logic and Bit Operations/Compare To Constant  relop===  const=1  OutDataTypeStr=boolean
  Logical Operator : Logic  Operator=OR  Inputs=20  AllPortsSameDT=off  OutDataTypeStr=boolean
  guzhang_rm : Outport
  wires:
  MCU2_3/1 -> Bus Selector/1
  Bus Selector/1 -> Compare To Constant/1  "<MCU2_3MotorStallingFault>"
  Bus Selector/2 -> Compare To Constant1/1  "<MCU2_3UdcDetectionFault>"
  Bus Selector/3 -> Compare To Constant2/1  "<MCU2_3TempSensorFault>"
  Bus Selector/4 -> Compare To Constant3/1  "<MCU2_3ActiveDischargingFault>"
  Bus Selector/5 -> Compare To Constant4/1  "<MCU2_3ldcSensorFault>"
  Bus Selector/6 -> Compare To Constant5/1  "<MCU2_3luSensorFault>"
  Bus Selector/7 -> Compare To Constant6/1  "<MCU2_3lvSensorFault>"
  Bus Selector/8 -> Compare To Constant7/1  "<MCU2_3FaultLevel>"
  Bus Selector/13 -> Compare To Constant12/1  "<MCU2_3IGBTFault>"
  Bus Selector/14 -> Compare To Constant13/1  "<MCU2_3MotorOverTemp>"
  Bus Selector/10 -> Compare To Constant9/1  "<MCU2_3CanCommunicationFault>"
  Bus Selector/16 -> Compare To Constant15/1  "<MCU2_3MotorOverSpeed>"
  Bus Selector/11 -> Compare To Constant10/1  "<MCU2_3MemoryFault>"
  Bus Selector/15 -> Compare To Constant14/1  "<MCU2_3ControllerOverTemp>"
  Bus Selector/12 -> Compare To Constant11/1  "<MCU2_3DownratingFault>"
  Bus Selector/9 -> Compare To Constant8/1  "<MCU2_3Controllerload>"
  Bus Selector/18 -> Compare To Constant17/1  "<MCU2_3UnderVoltage>"
  Bus Selector/20 -> Compare To Constant19/1  "<MCU2_3MotorOverLoad>"
  Bus Selector/19 -> Compare To Constant18/1  "<MCU2_3OverVoltage>"
  Bus Selector/17 -> Compare To Constant16/1  "<MCU2_3RotaryInverterFault>"
  Compare To Constant9/1 -> Logical Operator/10
  Compare To Constant12/1 -> Logical Operator/13
  Compare To Constant11/1 -> Logical Operator/12
  Compare To Constant15/1 -> Logical Operator/16
  Compare To Constant8/1 -> Logical Operator/9
  Compare To Constant10/1 -> Logical Operator/11
  Compare To Constant13/1 -> Logical Operator/14
  Compare To Constant14/1 -> Logical Operator/15
  Compare To Constant1/1 -> Logical Operator/2
  Compare To Constant17/1 -> Logical Operator/18
  Compare To Constant16/1 -> Logical Operator/17
  Compare To Constant18/1 -> Logical Operator/19
  Compare To Constant19/1 -> Logical Operator/20
  Compare To Constant3/1 -> Logical Operator/4
  Compare To Constant2/1 -> Logical Operator/3
  Compare To Constant6/1 -> Logical Operator/7
  Compare To Constant4/1 -> Logical Operator/5
  Compare To Constant5/1 -> Logical Operator/6
  Compare To Constant7/1 -> Logical Operator/8
  Compare To Constant/1 -> Logical Operator/1
  Logical Operator/1 -> guzhang_rm/1
